simulink model "Fuzzy_2409"  (R2016a)
settings: Solver=VariableStepAuto  StartTime=0.0  StopTime=10  FixedStep=0.0001  RelTol=1e-3
libraries: fuzblock x1
settings Model: Creator=USER  LastModifiedBy=USER

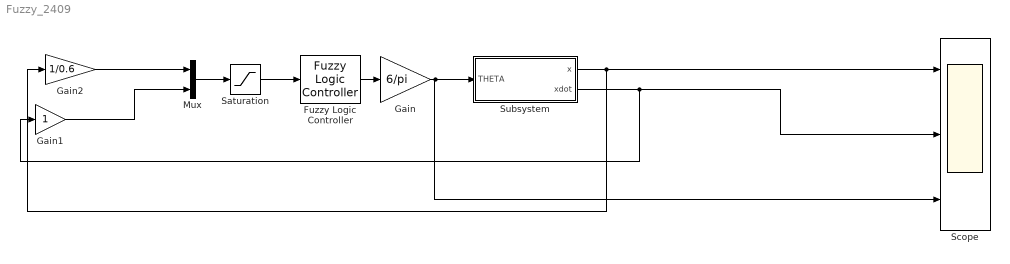
== system Fuzzy_2409 ==
  Fuzzy Logic Controller : fuzblock/Fuzzy Logic  Controller  fis=['EXPORT_BAI_1_BTVN3.fis']
  Gain : Gain  Gain=6/pi
  Gain1 : Gain
  Gain2 : Gain  Gain=1/0.6
  Mux : Mux  Inputs=2
  Saturation : Saturate  UpperLimit=1  LowerLimit=-1
  Scope : Scope  NumInputPorts=3
  Subsystem : Subsystem  mask{l=0.5, m=0.1, b=0.005, g=9.81, x0=0.1, xdot0=0.3, j=0.00005, r=0.02}
      mask prompts: l "chieu dai"; m "Khoi luong"; b "ma sat"; g "gia toc tt"; x0 "vi tri ban dau"; xdot0 "vt goc ban dau"; j "moment"; r "ban kinh bong"
  wires:
  Mux/1 -> Saturation/1
  Saturation/1 -> Fuzzy Logic Controller/1
  Fuzzy Logic Controller/1 -> Gain/1
  Gain/1 -> Scope/3, Subsystem/1(THETA)
  Subsystem/1("x ") -> Gain2/1, Scope/1
  Gain2/1 -> Mux/1
  Gain1/1 -> Mux/2
  Subsystem/2("xdot ") -> Gain1/1, Scope/2

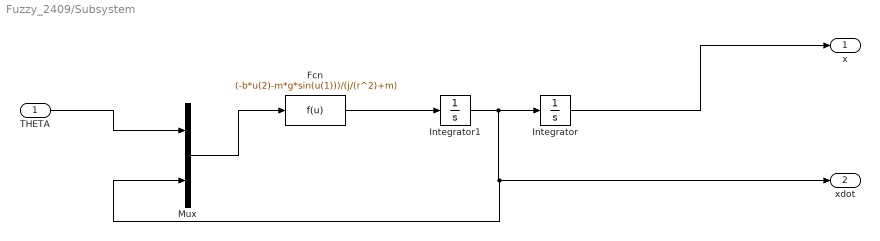
== system Fuzzy_2409/Subsystem ==
  THETA : Inport
  Fcn : Fcn  Expr=(-b*u(2)-m*g*sin(u(1)))/(j/(r^2)+m)
  Integrator : Integrator  InitialCondition=xdot0
  Integrator1 : Integrator  InitialCondition=x0
  Mux : Mux  Inputs=2
      settings: DisplayOption=signals
  "x " : Outport
  "xdot " : Outport  Port=2
  wires:
  Integrator/1 -> "x "/1
  Fcn/1 -> Integrator1/1
  THETA/1 -> Mux/1
  Mux/1 -> Fcn/1
  Integrator1/1 -> Mux/2, "xdot "/1, Integrator/1
